simulink model "Greenhouse_3rdPoint"  (R2024a)
settings: Solver=VariableStepAuto  StartTime=0.0  StopTime=10.0  RelTol=1e-3
values from neighbouring files (symbols this model uses):
  C_f1 = c_f * m_f1    (= 1846687500)    [init.m]
  C_f2 = c_f * m_f2    (= 492450000)    [init.m]
  kaf1 = t_t * Sm1_ext    (= 4731)    [init.m]
  kaf2 = t_t * Sm2_ext    (= 1311)    [init.m]
  kaf_int = t_t * Sm_int    (= 171)    [init.m]
  theta0_a = 100    [init.m]
  Ts = 1    [init.m]
  var_wf1 = 1    [init.m]
  var_wf2 = 1    [init.m]
settings Model: Creator=loren  LastModifiedBy=loren

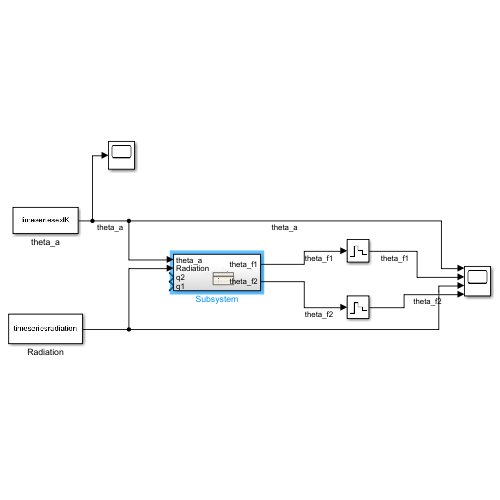
[thumbnail: Simulink's stored preview of the top-level diagram]
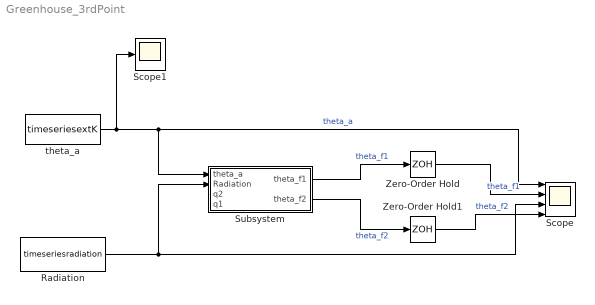
== system Greenhouse_3rdPoint ==
  Radiation : FromWorkspace  VariableName=timeseriesradiation  SampleTime=Ts
  Scope : Scope  NumInputPorts=4
  Scope1 : Scope
  Subsystem : Subsystem
  Zero-Order Hold : ZeroOrderHold  SampleTime=Ts
  Zero-Order Hold1 : ZeroOrderHold  SampleTime=Ts
  theta_a : FromWorkspace  VariableName=timeseriesextK  SampleTime=Ts
  wires:
  Subsystem/2(theta_f2) -> Zero-Order Hold1/1  "theta_f2"
  Radiation/1 -> Scope/3, Subsystem/2(Radiation)
  Zero-Order Hold1/1 -> Scope/4  "theta_f2"
  Subsystem/1(theta_f1) -> Zero-Order Hold/1  "theta_f1"
  Zero-Order Hold/1 -> Scope/2  "theta_f1"
  theta_a/1 -> Scope1/1, Scope/1, Subsystem/1(theta_a)  "theta_a"

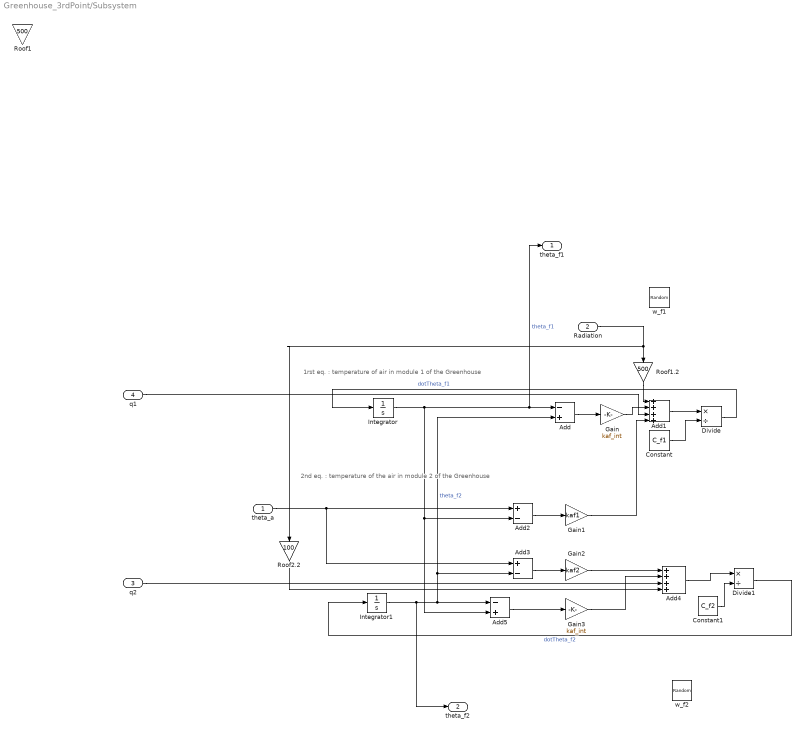
== system Greenhouse_3rdPoint/Subsystem ==
  note: 2nd eq. : temperature of the air in module 2 of the Greenhouse
  note: 1rst eq. : temperature of air in module 1 of the Greenhouse
  theta_a : Inport
  Radiation : Inport  Port=2
  q2 : Inport  Port=3
  q1 : Inport  Port=4
  Add : Sum  Inputs=-+
  Add1 : Sum  Inputs=++++
  Add2 : Sum  Inputs=+-
  Add3 : Sum  Inputs=+-
  Add4 : Sum  Inputs=++++
  Add5 : Sum  Inputs=-+
  Constant : Constant  Value=C_f1
  Constant1 : Constant  Value=C_f2
  Divide : Product  Inputs=*/
  Divide1 : Product  Inputs=*/
  Gain : Gain  Gain=kaf_int
  Gain1 : Gain  Gain=kaf1
  Gain2 : Gain  Gain=kaf2
  Gain3 : Gain  Gain=kaf_int
  Integrator : Integrator  InitialCondition=theta0_a
  Integrator1 : Integrator  InitialCondition=theta0_a
  Roof1 : Gain  Gain=500
  Roof1.2 : Gain  Gain=500
  Roof2.2 : Gain  Gain=100
  w_f1 : RandomNumber  Variance=var_wf1  SampleTime=Ts
  w_f2 : RandomNumber  Variance=var_wf2  SampleTime=Ts
  theta_f1 : Outport
  theta_f2 : Outport  Port=2
  wires:
  Add/1 -> Gain/1
  Gain1/1 -> Add1/4
  Add5/1 -> Gain3/1
  Add4/1 -> Divide1/1
  Integrator1/1 -> theta_f2/1, Add3/2, Add/2, Add5/1  "theta_f2"
  Divide1/1 -> Integrator1/1  "dotTheta_f2"
  Gain/1 -> Add1/2
  Radiation/1 -> Roof2.2/1, Roof1.2/1
  Constant/1 -> Divide/2
  Add1/1 -> Divide/1
  Add2/1 -> Gain1/1
  Add3/1 -> Gain2/1
  theta_a/1 -> Add3/1, Add2/1
  Integrator/1 -> Add5/2, Add2/2, theta_f1/1, Add/1  "theta_f1"
  Divide/1 -> Integrator/1  "dotTheta_f1"
  Gain3/1 -> Add4/2
  Gain2/1 -> Add4/1
  Constant1/1 -> Divide1/2
  Roof1.2/1 -> Add1/1
  Roof2.2/1 -> Add4/4
  q1/1 -> Add1/3
  q2/1 -> Add4/3
